simulink model "HexrotorDynamicModel_matlab2010"  (Simulink 7.6)
settings: Solver=ode3  SolverMode=SingleTasking  StartTime=0.0  StopTime=20  FixedStep=0.0005  RelTol=1e-3
values from neighbouring files (symbols this model uses):
  alpha = pi/180 * 13.6    (= 0.237364778271)    [IdealParameter.m]    (also in ParLuk11.m = deg2rad(13.6); Parameter.m = [-alpha_i;alpha_i;-alpha_i;alpha_i;-alpha_i;alpha_i]; ParameterIdeal.m = [-alpha_i;alpha_i;-alpha_i;alpha_i;-alpha_i;alpha_i]; ParameterVIVE.m = [alpha_i;-alpha_i;alpha_i;-alpha_i;alpha_i;-alpha_i])
  alpha_0 = alpha    (= 0.237364778271)    [IdealParameter.m]    (also in Parameter.m = alpha; ParameterIdeal.m = alpha*1.01; ParameterVIVE.m = alpha*1.01; ParameterVO.m = alpha*1.01)
  angular_noise = 0    [IdealParameter.m]    (also in Parameter.m = 0.5; ParameterIdeal.m; ParameterVIVE.m; ParameterVO.m)
  b = 1.1e-06    [IdealParameter.m]    (also in ParLuk11.m = 1.14e-07; Parameter.m = 8.944e-07; ParameterIdeal.m; ParameterVIVE.m)
  b_0 = b*1.15    (= 1.265e-06)    [IdealParameter.m]    (also in Parameter.m = 8.944e-07; ParameterIdeal.m; ParameterVIVE.m; ParameterVO.m)
  beta = 0    [IdealParameter.m]    (also in ParLuk11.m; Parameter.m = [beta_i; beta_i; beta_i; beta_i; beta_i; beta_i]; ParameterIdeal.m = [beta_i; beta_i; beta_i; beta_i; beta_i; beta_i]; ParameterVIVE.m = [beta_i; beta_i; beta_i; beta_i; beta_i; beta_i])
  beta_0 = beta    (= 0)    [IdealParameter.m]    (also in Parameter.m = beta; ParameterIdeal.m = beta*0.99; ParameterVIVE.m = beta*0.99; ParameterVO.m = beta*0.99)
  eta = 1    [Controllability.m]    (also in IdealParameter.m = 75; Parameter.m = 2; ParameterIdeal.m = 40; ParameterVIVE.m = 10)
  eta_rot = 50    [IdealParameter.m]    (also in Parameter.m = 2; ParameterIdeal.m = 20; ParameterVIVE.m = 5; ParameterVO.m = 2)
  g = 9.81    [IdealParameter.m]    (also in ParLuk11.m; Parameter.m; ParameterIdeal.m; ParameterVIVE.m)
  g_0 = g*0.99    (= 9.7119)    [IdealParameter.m]    (also in Parameter.m = 9.81; ParameterIdeal.m = 9.81; ParameterVIVE.m = 9.81; ParameterVO.m = 9.81)
  IB = [Ixx 0 0; 0 Iyy 0; 0 0 Izz]    [IdealParameter.m]    (also in ParLuk11.m; Parameter.m; ParameterIdeal.m; ParameterVIVE.m)
  IB_0 = IB*1.07    [IdealParameter.m]    (also in Parameter.m = IB; ParameterIdeal.m; ParameterVIVE.m; ParameterVO.m)
  k = 5.6e-05    [IdealParameter.m]    (also in ParLuk11.m = 2.98e-06; Parameter.m = 4.472e-05; ParameterIdeal.m; ParameterVIVE.m = 5.13e-05)
  K_0 = Ts/(T_rotor_0+Ts)    (= 0.0384615384615)    [IdealParameter.m]    (also in Parameter.m = 0.230769230769; ParameterIdeal.m; ParameterVIVE.m = 0.0350877192982; ParameterVO.m = 0.214285714286)
  k_0 = k*1.16    (= 6.496e-05)    [IdealParameter.m]    (also in Parameter.m = 4.472e-05; ParameterIdeal.m; ParameterVIVE.m = 5.9508e-05; ParameterVO.m)
  K_d = diag([5,5,5,2,2,2])    [ParLuk11.m]
  K_p1 = 10*eye(3)    [ParLuk11.m]
  k_p2 = 3    [ParLuk11.m]
  K_P_1 = 15*eye(3)    [IdealParameter.m]    (also in Parameter.m = 2*eye(3); ParameterIdeal.m; ParameterVIVE.m = 10*eye(3); ParameterVO.m = 2*eye(3))
  K_P_2 = 50*eye(3)    [IdealParameter.m]    (also in Parameter.m = 4*eye(3); ParameterIdeal.m; ParameterVIVE.m = 10*eye(3); ParameterVO.m = 4*eye(3))
  K_P_3 = 60*eye(3)    [IdealParameter.m]    (also in Parameter.m = 6*eye(3); ParameterIdeal.m; ParameterVIVE.m = 10*eye(3); ParameterVO.m = 6*eye(3))
  K_P_D = 30*eye(3)    [IdealParameter.m]    (also in ParLuk11.m = 10*eye(3); Parameter.m = 5*eye(3); ParameterIdeal.m; ParameterVIVE.m = 15*eye(3))
  K_P_I = 100*eye(3)    [IdealParameter.m]    (also in ParLuk11.m = 10*eye(3); Parameter.m = 10*eye(3); ParameterIdeal.m = 80*eye(3); ParameterVIVE.m)
  K_P_P = 100*eye(3)    [IdealParameter.m]    (also in ParLuk11.m = 20*eye(3); Parameter.m = 10*eye(3); ParameterIdeal.m = 130*eye(3); ParameterVIVE.m)
  K_R_1 = 40*eye(3)    [IdealParameter.m]    (also in Parameter.m = 2*eye(3); ParameterIdeal.m; ParameterVIVE.m = 10*eye(3); ParameterVO.m = 2*eye(3))
  K_R_2 = 100*eye(3)    [IdealParameter.m]    (also in Parameter.m = 4*eye(3); ParameterIdeal.m; ParameterVIVE.m = 10*eye(3); ParameterVO.m = 4*eye(3))
  K_R_3 = 50*eye(4)    [IdealParameter.m]    (also in Parameter.m = 6*eye(4); ParameterIdeal.m; ParameterVIVE.m = 10*eye(4); ParameterVO.m = 6*eye(4))
  K_R_D = 30*eye(3)    [IdealParameter.m]    (also in ParLuk11.m = 10*eye(3); Parameter.m = 5*eye(3); ParameterIdeal.m; ParameterVIVE.m = 15*eye(3))
  K_R_I = 100*eye(3)    [IdealParameter.m]    (also in ParLuk11.m = 10*eye(3); Parameter.m = 10*eye(3); ParameterIdeal.m = 80*eye(3); ParameterVIVE.m)
  K_R_P = 100*eye(3)    [IdealParameter.m]    (also in ParLuk11.m = 20*eye(3); Parameter.m = 10*eye(3); ParameterIdeal.m = 130*eye(3); ParameterVIVE.m)
  L = 0.4    [IdealParameter.m]    (also in ParLuk11.m = 1; Parameter.m; ParameterIdeal.m; ParameterVIVE.m = 0.6)
  L_0 = L*1.02    (= 0.408)    [IdealParameter.m]    (also in Parameter.m = 0.4; ParameterIdeal.m; ParameterVIVE.m = 0.612; ParameterVO.m)
  lambda = 10    [IdealParameter.m]    (also in Parameter.m = 3; ParameterIdeal.m = 5; ParameterVIVE.m = 5; ParameterVO.m = 3)
  lambda_rot = 10    [IdealParameter.m]    (also in Parameter.m = 3; ParameterIdeal.m; ParameterVIVE.m = 5; ParameterVO.m = 3)
  m = 1    [Controllability.m]    (also in IdealParameter.m = 2.5; ParLuk11.m = 0.6; Parameter.m = 4.85; ParameterIdeal.m = 4.85)
  M = 50    [IdealParameter.m]    (also in Parameter.m = 6; ParameterIdeal.m = 100; ParameterVIVE.m = 5; ParameterVO.m = 6)
  m_0 = m*1.03    (= 2.575)    [IdealParameter.m]    (also in Parameter.m = 4.85; ParameterIdeal.m = 4.9955; ParameterVIVE.m = 4.52994; ParameterVO.m = 4.9955)
  M_rot = 50    [IdealParameter.m]    (also in Parameter.m = 6; ParameterIdeal.m = 15; ParameterVIVE.m = 1; ParameterVO.m = 6)
  omega_noise = 0    [IdealParameter.m]    (also in Parameter.m = sqrt(2)*angular_noise/Ts * pi/180; ParameterIdeal.m; ParameterVIVE.m; ParameterVO.m)
  p_noise = 0    [IdealParameter.m]    (also in Parameter.m = 0.001; ParameterIdeal.m; ParameterVIVE.m; ParameterVO.m)
  T_delay = 0    [IdealParameter.m]    (also in Parameter.m = 0.1; ParameterIdeal.m; ParameterVIVE.m = 0.04; ParameterVO.m = 0.1)
  T_rotor = 0.1    [IdealParameter.m]    (also in Parameter.m; ParameterIdeal.m; ParameterVIVE.m; ParameterVO.m)
  Ts = 1/250    (= 0.004)    [IdealParameter.m]    (also in Parameter.m = 0.03; ParameterIdeal.m; ParameterVIVE.m; ParameterVO.m = 0.03)
  v_noise = 0    [IdealParameter.m]    (also in Parameter.m = sqrt(2)*p_noise/Ts; ParameterIdeal.m; ParameterVIVE.m; ParameterVO.m)
  z_p_0 = T_rotor_0/(T_rotor_0+Ts)    (= 0.961538461538)    [IdealParameter.m]    (also in Parameter.m = 0.769230769231; ParameterIdeal.m; ParameterVIVE.m = 0.964912280702; ParameterVO.m = 0.785714285714)
undefined symbols (not defined in the file or in its folder): DiscIntNeverNeededParam, k_ad, k_ap, k_pd, k_pp, k_z
libraries: vrlib x8, simulink x7, dspmtrx3 x3
(part 1 of 3)
settings Model: Creator=jan  LastModifiedBy=Jan  CovMetricSettings=dwe  CovHtmlReporting=off  covSaveCumulativeToWorkspaceVar=off  CovSaveSingleToWorkspaceVar=off  CovExternalEMLEnable=on
settings DataIOCC: LimitDataPoints=off  SaveFormat=StructureWithTime
settings OptimizationCC: ExpressionDepthLimit=128
settings DebuggingCC: UnderspecifiedInitializationDetection=Simplified  MergeDetectMultiDrivingBlocksExec=error  SolverPrmCheckMsg=none  FcnCallInpInsideContextMsg=Enable All  StateNameClashWarn=none  SFUnexpectedBacktrackingDiag=error  SFNoUnconditionalDefaultTransitionDiag=error
settings HardwareCC: ProdBitPerPointer=64  ProdLargestAtomicFloat=Float  ProdIntDivRoundTo=Zero  ProdEndianess=LittleEndian  ProdHWDeviceType=Specified
settings CodeAppCC: CustomSymbolStrType=$N$R$M_T
settings GRTTargetCC: TargetFunctionLibrary=C99 (ISO)  GeneratePreprocessorConditionals=Use local settings

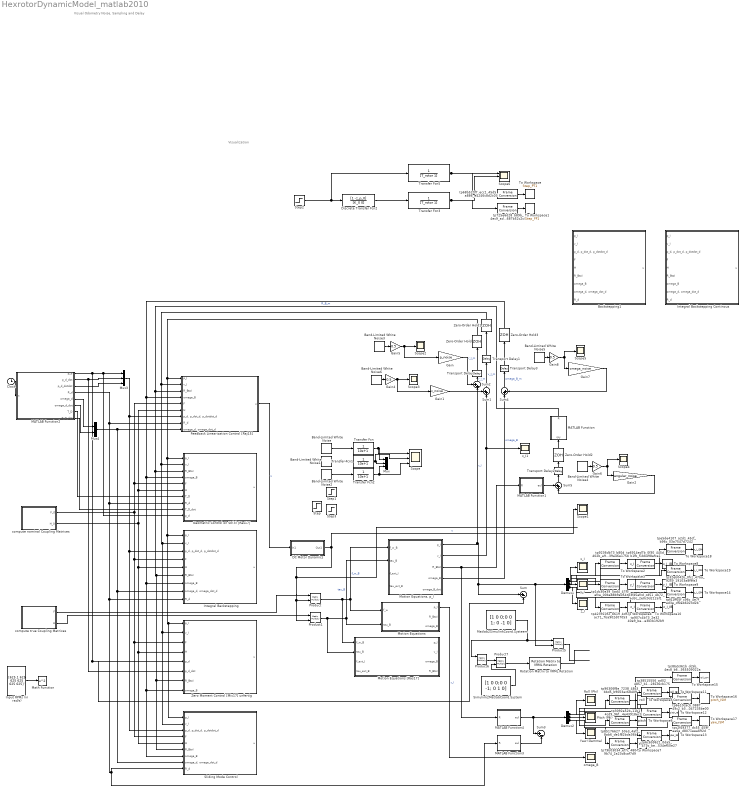
== system HexrotorDynamicModel_matlab2010 ==
  note: Visual Odometry Noise, Sampling and Delay
  note: Visualization
  Backstepping1 : Subsystem
  Band-Limited White Noise : simulink/Sources/Band-Limited White Noise  Cov=10  Ts=0.1  seed=[28341]  VectorParams1D=off
  Band-Limited White Noise1 : simulink/Sources/Band-Limited White Noise  Cov=10  Ts=0.1  seed=[23342]  VectorParams1D=off
  Band-Limited White Noise2 : simulink/Sources/Band-Limited White Noise  Cov=10  Ts=0.1  seed=[23441]  VectorParams1D=off
  Band-Limited White Noise3 : simulink/Sources/Band-Limited White Noise  Cov=[0.01; 0.01; 0.01]  Ts=Ts  seed=[22352; 29655; 12541]  VectorParams1D=off
  Band-Limited White Noise4 : simulink/Sources/Band-Limited White Noise  Cov=[0.01; 0.01; 0.01]  Ts=Ts  seed=[11351; 22653; 52546]  VectorParams1D=off
  Band-Limited White Noise5 : simulink/Sources/Band-Limited White Noise  Cov=[0.01; 0.01; 0.01]  Ts=Ts  seed=[12451; 82653; 82546]  VectorParams1D=off
  Band-Limited White Noise6 : simulink/Sources/Band-Limited White Noise  Cov=[0.01; 0.01; 0.01]  Ts=Ts  seed=[22351; 29653; 12546]  VectorParams1D=off
  Clock : Clock
  "DC Motor Dynamics " : Subsystem  TreatAsAtomicUnit=on
  Demux1 : Demux  Outputs=3
  Demux2 : Demux  Outputs=3
  Discrete Transfer Fcn2 : DiscreteTransferFcn  Numerator=[1 -z_p_0]  Denominator=[K_0 0]  InitialStates=550  SampleTime=Ts
  Feedback Linearization Control [Raj15] : Subsystem
  Gain : Gain  Gain=p_noise
  Gain1 : Gain  Gain=v_noise
  Gain2 : Gain  Gain=angular_noise
  Gain{4..6,8} (4 alike) : Gain  Gain=0.5
  Gain7 : Gain  Gain=omega_noise
  Geometric Control on SE(3) [Ras17] : Subsystem
  Input RPMs (in rad/s) : Constant  Value=[625.1 625 625 625 625 625]'  VectorParams1D=off
  Integral Backstepping : Subsystem
  "Integral Backstepping Continous " : Subsystem
  MATLAB Function : Stateflow chart  TreatAsAtomicUnit=on
      settings: PermitHierarchicalResolution=ParametersOnly
  MATLAB Function1 : Stateflow chart  TreatAsAtomicUnit=on
      settings: PermitHierarchicalResolution=ParametersOnly
  MATLAB Function2 : Stateflow chart  TreatAsAtomicUnit=on
      settings: PermitHierarchicalResolution=ParametersOnly
  MATLAB Function3 : Stateflow chart  TreatAsAtomicUnit=on
      settings: PermitHierarchicalResolution=ParametersOnly
  MATLAB Function4 : Stateflow chart  TreatAsAtomicUnit=on
      settings: PermitHierarchicalResolution=ParametersOnly
  Math Function : Math  Operator=square  SaturateOnIntegerOverflow=on
  "Matlab2SimulinkCoord.Systeem " : Constant  Value=[1 0 0;0 0 1; 0 -1 0]  VectorParams1D=off
  Motion Equations : Subsystem
  Motion Equations [Ras17] : Subsystem
  "Motion Equations, p_I" : Subsystem
  Mux : Mux  Inputs=3
  Mux3 : Mux  Inputs=3
  Mux4 : Mux  Inputs=2
  Pitch (Psi) : Scope
      settings: TimeRange=auto  MaxDataPoints=5000  SaveToWorkspace=off  YMin=-3.22277  YMax=12.55112  SampleTime=-1
  Product{,1,5..7} (5 alike) : Product  Multiplication=Matrix(*)
  Roll (Phi) : Scope
      settings: TimeRange=auto  MaxDataPoints=5000  SaveToWorkspace=off  SaveName=ScopeData2  YMin=-4.01127  YMax=16.26235  SampleTime=-1
  Rotation Matrix to VRML Rotation : vrlib/Utilities/Rotation Matrix to VRML Rotation  maxzero=1e-12
  Scope : Scope  NumInputPorts=3
      settings: TimeRange=auto  MaxDataPoints=5000  SaveToWorkspace=off  YMin=-1.78932~-5~-5  YMax=1.08657~5~5  SampleTime=-1
  Scope{1..5} (5 alike) : Scope
      Scope1 settings: TimeRange=auto  MaxDataPoints=5000  SaveToWorkspace=off  YMin=-244096.59135  YMax=3111530.80524  SampleTime=-1
      Scope2 settings: TimeRange=auto  MaxDataPoints=5000  SaveToWorkspace=off  YMin=-1.60588  YMax=1.50821  SampleTime=-1
      Scope3 settings: TimeRange=auto  MaxDataPoints=5000  SaveToWorkspace=off  SaveName=ScopeData2  YMin=-1.55633  YMax=1.34059  SampleTime=-1
      Scope4 settings: TimeRange=auto  MaxDataPoints=5000  SaveToWorkspace=off  SaveName=ScopeData2  YMin=-1.57808  YMax=1.44255  SampleTime=-1
      Scope5 settings: TimeRange=auto  MaxDataPoints=5000  SaveToWorkspace=off  SaveName=ScopeData3  YMin=-3.75052  YMax=3.91407  SampleTime=-1
  Scope6 : Scope  NumInputPorts=3
      settings: TimeRange=auto  MaxDataPoints=5000  SaveToWorkspace=off  YMin=-0.61685~-5~-5  YMax=2.28631~5~5  SampleTime=-1
  "Simulink2MatlabCoord.System " : Constant  Value=[1 0 0;0 0 -1; 0 1 0]  VectorParams1D=off
  Sliding Mode Control : Subsystem
  Step : Step  Time=0.1  Before=[6,0,6]'  After=[0,0,0]'  SampleTime=0  VectorParams1D=off
  Step1 : Step  Before=[0;0;0]  After=[10;1;1]  SampleTime=0  VectorParams1D=off
  Step2 : Step  SampleTime=0
  Step3 : Step  Before=[0;0;0]  After=[5;1;1]  SampleTime=0  VectorParams1D=off
  Sum : Sum  Inputs=|+-
  Sum1 : Sum  Inputs=++|
  Sum2 : Sum  Inputs=++|
  Sum3 : Sum  Inputs=|+-
  Sum4 : Sum  Inputs=|++
  Sum5 : Sum  Inputs=++|
  To Workspace : ToWorkspace  VariableName=Step_PT1  SampleTime=Ts
  To Workspace1 : ToWorkspace  VariableName=Step_FF1  SampleTime=Ts
  To Workspace10 : ToWorkspace  VariableName=z_I_IB  SampleTime=Ts
  To Workspace11 : ToWorkspace  VariableName=roll_IB  SampleTime=Ts
  To Workspace12 : ToWorkspace  VariableName=pitch_IB  SampleTime=Ts
  To Workspace13 : ToWorkspace  VariableName=yaw_IB  SampleTime=Ts
  To Workspace14 : ToWorkspace  VariableName=z_I_ISM  SampleTime=Ts
  To Workspace15 : ToWorkspace  VariableName=roll_ISM  SampleTime=Ts
  To Workspace16 : ToWorkspace  VariableName=pitch_ISM  SampleTime=Ts
  To Workspace17 : ToWorkspace  VariableName=yaw_ISM  SampleTime=Ts
  To Workspace18 : ToWorkspace  VariableName=x_I_ISM  SampleTime=Ts
  To Workspace19 : ToWorkspace  VariableName=y_I_ISM  SampleTime=Ts
  To Workspace2 : ToWorkspace  VariableName=x_I  SampleTime=Ts
  To Workspace3 : ToWorkspace  VariableName=y_I  SampleTime=Ts
  To Workspace4 : ToWorkspace  VariableName=z_I  SampleTime=Ts
  To Workspace5 : ToWorkspace  VariableName=roll  SampleTime=Ts
  To Workspace6 : ToWorkspace  VariableName=pitch  SampleTime=Ts
  To Workspace7 : ToWorkspace  VariableName=yaw  SampleTime=Ts
  To Workspace8 : ToWorkspace  VariableName=x_I_IB  SampleTime=Ts
  To Workspace9 : ToWorkspace  VariableName=y_I_IB  SampleTime=Ts
  Transfer Fcn : TransferFcn  Denominator=[10 1]
  Transfer Fcn1 : TransferFcn  Denominator=[10 1]
  Transfer Fcn2 : TransferFcn  Denominator=[10 1]
  Transfer Fcn3 : TransferFcn  Denominator=[T_rotor 1]
  Transfer Fcn5 : TransferFcn  Denominator=[T_rotor 1]
  Transport Delay{,1..3} (4 alike) : TransportDelay  DelayTime=T_delay  InitialOutput=[0;0;0]
  Yaw (Gamma) : Scope
      settings: TimeRange=auto  MaxDataPoints=5000  SaveToWorkspace=off  SaveName=ScopeData3  YMin=-2.81636  YMax=2.98602  SampleTime=-1
  Zero Moment Control [Mic17] unfertig : Subsystem
  Zero-Order Hold : ZeroOrderHold  SampleTime=0.02
  Zero-Order Hold1 : ZeroOrderHold  SampleTime=0.01
  Zero-Order Hold2 : ZeroOrderHold  SampleTime=Ts
  Zero-Order Hold3 : ZeroOrderHold  SampleTime=0.01
  compute nominal Coupling Matrices : Subsystem
  compute true Coupling Matrices : Subsystem
  omega_B : Scope
      settings: TimeRange=auto  LimitDataPoints=on  MaxDataPoints=5000  SaveToWorkspace=off  SaveName=ScopeData4  YMin=-0.00000000000000000  YMax=0.00000000000000017  SampleTime=-1  DataFormat=Array
  tp1dc30e39_5ad4_47f3_afca_00ba88b9e054 : FrameConversion  InheritSamplingMode=off  OutFrame=Sample-based
  tp3092a52b_11b1_4cd9_96f5_a04e43918ec3 : FrameConversion  InheritSamplingMode=off  OutFrame=Sample-based
  tp32eb042b_0fcc_47ba_92c9_19103a8f9fa3 : FrameConversion  InheritSamplingMode=off  OutFrame=Sample-based
  tp38515556_ad02_4857_b18b_e4281c6cb175 : FrameConversion  InheritSamplingMode=off  OutFrame=Sample-based
  tp38a5361b_dc5b_4ec8_b600_69955509022a : FrameConversion  InheritSamplingMode=off  OutFrame=Sample-based
  tp3f45afcd_cd51_4b72_ad3c_2e0c0d212af1 : FrameConversion  InheritSamplingMode=off  OutFrame=Sample-based
  tp4239105c_b619_4df0_ac71_7ba902d07053 : FrameConversion  InheritSamplingMode=off  OutFrame=Sample-based
  tp68b520f7_ecc1_45d5_a886_e4246c8d2c03 : FrameConversion  InheritSamplingMode=off  OutFrame=Sample-based
  tp6914ed7b_0f30_445d_b1fb_f1bb498efca1 : FrameConversion  InheritSamplingMode=off  OutFrame=Sample-based
  tp6c6b9621_0da5_473c_be95_13534ef50e27 : FrameConversion  InheritSamplingMode=off  OutFrame=Sample-based
  tp6e10cacb_0887_49c2_b351_a1047235be00 : FrameConversion  InheritSamplingMode=off  OutFrame=Sample-based
  tp725e6d28_b89b_4ec9_adef_fa687b52c2c8 : FrameConversion  InheritSamplingMode=off  OutFrame=Sample-based
  tp79b03034_ef7c_4804_9b74_2a23c8caf7d9 : FrameConversion  InheritSamplingMode=off  OutFrame=Sample-based
  tp85176627_50a3_4af2_8ab6_de1f82bda36b : FrameConversion  InheritSamplingMode=off  OutFrame=Sample-based
  tp907c4b73_2e32_40e9_be19_e2e3bcb192b9 : FrameConversion  InheritSamplingMode=off  OutFrame=Sample-based
  tp9236db73_b80d_402b_a970_1639a46e175b : FrameConversion  InheritSamplingMode=off  OutFrame=Sample-based
  tp96306f8e_7238_48c3_bbd5_b9003ac68409 : FrameConversion  InheritSamplingMode=off  OutFrame=Sample-based
  tpc2f49377_dc55_459f_aa6e_d8071eeab92d : FrameConversion  InheritSamplingMode=off  OutFrame=Sample-based
  tpe5de4107_a2d1_45cf_b96c_03a7547d7242 : FrameConversion  InheritSamplingMode=off  OutFrame=Sample-based
  tpf41ff05f_c96c_4e7f_ad3e_df0ab6023d2b : FrameConversion  InheritSamplingMode=off  OutFrame=Sample-based
  x_I : Scope
      settings: TimeRange=auto  MaxDataPoints=5000  SaveToWorkspace=off  SaveName=ScopeData6  YMin=-0.2003  YMax=1.67814  SampleTime=-1
  x_I1 : Scope
      settings: TimeRange=auto  MaxDataPoints=5000  SaveToWorkspace=off  YMin=-0.67724  YMax=1.12529  SampleTime=-1
  y_I : Scope
      settings: TimeRange=auto  MaxDataPoints=5000  SaveToWorkspace=off  SaveName=ScopeData7  YMin=-0.14547  YMax=1.20694  SampleTime=-1
  z_I : Scope
      settings: TimeRange=auto  MaxDataPoints=5000  SaveToWorkspace=off  SaveName=ScopeData  YMin=-0.17063  YMax=0.10776  SampleTime=-1
  wires:
  Product6/1 -> Product7/1
  Product5/1 -> ?
  Demux2/2 -> tp3092a52b_11b1_4cd9_96f5_a04e43918ec3/1, tp6e10cacb_0887_49c2_b351_a1047235be00/1, Pitch (Psi)/1, tp85176627_50a3_4af2_8ab6_de1f82bda36b/1
  Input RPMs (in rad/s)/1 -> Math Function/1
  Transport Delay/1 -> Zero-Order Hold/1  "r_I_m"
  Demux1/3 -> tp907c4b73_2e32_40e9_be19_e2e3bcb192b9/1, tpf41ff05f_c96c_4e7f_ad3e_df0ab6023d2b/1, z_I/1, tp4239105c_b619_4df0_ac71_7ba902d07053/1
  Demux1/1 -> tpe5de4107_a2d1_45cf_b96c_03a7547d7242/1, tp9236db73_b80d_402b_a970_1639a46e175b/1, x_I/1, tp6914ed7b_0f30_445d_b1fb_f1bb498efca1/1
  "DC Motor Dynamics "/1(Out1) -> Product1/2, Product/2, Scope1/1  "u"
  Demux1/2 -> tp32eb042b_0fcc_47ba_92c9_19103a8f9fa3/1, tp1dc30e39_5ad4_47f3_afca_00ba88b9e054/1, y_I/1, tp3f45afcd_cd51_4b72_ad3c_2e0c0d212af1/1
  Rotation Matrix to VRML Rotation/1 -> ?
  Demux2/1 -> tp38515556_ad02_4857_b18b_e4281c6cb175/1, tp38a5361b_dc5b_4ec8_b600_69955509022a/1, Roll (Phi)/1, tp96306f8e_7238_48c3_bbd5_b9003ac68409/1
  "Matlab2SimulinkCoord.Systeem "/1 -> Product6/1, Product5/1
  Product7/1 -> Rotation Matrix to VRML Rotation/1
  "Simulink2MatlabCoord.System "/1 -> Product7/2
  MATLAB Function/1(R) -> Geometric Control on SE(3) [Ras17]/3("R_BtoI "), Sliding Mode Control/6(R_BtoI), Zero Moment Control [Mic17] unfertig/7(R_BtoI), Integral Backstepping/6(R_BtoI), Feedback Linearization Control [Raj15]/3("R_BtoI ")  "R_B_m"
  Sum4/1 -> Transport Delay3/1  "omega_B_m"
  Motion Equations/1(p_I) -> omega_B/1  "r_I"
  compute nominal Coupling Matrices/1(F_0) -> Sliding Mode Control/4(F), Zero Moment Control [Mic17] unfertig/3(F), Integral Backstepping/4(F), Geometric Control on SE(3) [Ras17]/5(F), Feedback Linearization Control [Raj15]/5(F)
  Product/1 -> Motion Equations [Ras17]/1("f_w_B "), Motion Equations/1("f_w "), "Motion Equations, p_I"/1("f_w_B ")  "f_w_B"
  compute nominal Coupling Matrices/2("H_0 ") -> Zero Moment Control [Mic17] unfertig/4(H), Sliding Mode Control/5(H), Integral Backstepping/5(H), Geometric Control on SE(3) [Ras17]/6(H), Feedback Linearization Control [Raj15]/6(H)
  Product1/1 -> Motion Equations [Ras17]/2(tau_B), "Motion Equations, p_I"/2(tau_B), Motion Equations/2(tau_B)  "tau_B"
  Clock/1 -> MATLAB Function2/1(t)
  MATLAB Function2/3(p_d_dotdot) -> Mux3/3
  MATLAB Function2/2(p_d_dot) -> Zero Moment Control [Mic17] unfertig/6(p_d_dot), Mux3/2
  MATLAB Function2/1(p_d) -> Sum/2, Zero Moment Control [Mic17] unfertig/5(p_d), Geometric Control on SE(3) [Ras17]/10(p_d), Mux3/1
  MATLAB Function2/6(omega_d_dot) -> Mux4/2
  Band-Limited White Noise/1 -> Transfer Fcn/1
  Transfer Fcn/1 -> Scope/1, Mux/1
  Transfer Fcn2/1 -> Scope/3, Mux/3
  Band-Limited White Noise1/1 -> Transfer Fcn1/1
  Band-Limited White Noise2/1 -> Transfer Fcn2/1
  Transfer Fcn1/1 -> Scope/2, Mux/2
  Mux3/1 -> Sliding Mode Control/3("p_d, p_dot_d, p_dotdot_d"), Integral Backstepping/3("p_d, p_dot_d, p_dotdot_d"), Feedback Linearization Control [Raj15]/7("p_d, p_dot_d, p_dotdot_d")
  MATLAB Function2/4(R_d) -> MATLAB Function3/1(R), Sliding Mode Control/9(R_d), Integral Backstepping/9(R_d), Geometric Control on SE(3) [Ras17]/8(R_d), Feedback Linearization Control [Raj15]/8(R_d)
  MATLAB Function2/5(omega_d) -> Mux4/1
  Mux4/1 -> Sliding Mode Control/8("omega_d, omega_dot_d"), Integral Backstepping/8("omega_d, omega_dot_d"), Feedback Linearization Control [Raj15]/9("omega_d, omega_dot_d")
  MATLAB Function2/7(T_D) -> Geometric Control on SE(3) [Ras17]/7(T_D)
  MATLAB Function2/8(T_D_dot) -> Geometric Control on SE(3) [Ras17]/9(T_D_dot)
  compute true Coupling Matrices/1(F) -> Product/1
  compute true Coupling Matrices/2(H) -> Product1/1
  "Motion Equations, p_I"/1(p_I) -> Sum/1, Demux1/1, Product5/2, Sum2/2  "r_I"
  "Motion Equations, p_I"/2(v_I) -> x_I1/1, Sum1/2
  "Motion Equations, p_I"/3(R_BtoI) -> MATLAB Function4/1(R), MATLAB Function1/1(R)
  "Motion Equations, p_I"/4(omega_B) -> Sum4/1  "omega_B"
  Gain/1 -> Sum2/1
  Band-Limited White Noise3/1 -> Gain5/1
  Gain4/1 -> Gain1/1, Scope3/1
  Gain1/1 -> Sum1/1
  Sum2/1 -> Transport Delay/1  "r_I_m"
  Transport Delay1/1 -> Zero-Order Hold1/1
  Sum1/1 -> Transport Delay1/1  "v_I_m"
  Zero-Order Hold/1 -> Geometric Control on SE(3) [Ras17]/1("p_I "), Sliding Mode Control/1(p_I), Zero Moment Control [Mic17] unfertig/1(p_I), Integral Backstepping/1(p_I), Feedback Linearization Control [Raj15]/1("p_I ")
  Zero-Order Hold1/1 -> Sliding Mode Control/2(v_I), Zero Moment Control [Mic17] unfertig/2(v_I), Integral Backstepping/2(v_I), Geometric Control on SE(3) [Ras17]/2(v_I), Feedback Linearization Control [Raj15]/2(v_I)
  MATLAB Function1/1(eul) -> Sum5/1
  Gain6/1 -> Scope4/1, Gain2/1
  Sum5/1 -> Transport Delay2/1
  Gain2/1 -> Sum5/2
  Zero-Order Hold2/1 -> MATLAB Function/1(rpy)
  Transport Delay2/1 -> Zero-Order Hold2/1
  Transport Delay3/1 -> Zero-Order Hold3/1
  Zero-Order Hold3/1 -> Sliding Mode Control/7(omega_B), Zero Moment Control [Mic17] unfertig/8(omega_B), Integral Backstepping/7(omega_B), Geometric Control on SE(3) [Ras17]/4(omega_B), Feedback Linearization Control [Raj15]/4(omega_B)
  Feedback Linearization Control [Raj15]/1(u) -> "DC Motor Dynamics "/1(In1)  "u"
  Band-Limited White Noise6/1 -> Gain4/1
  Gain5/1 -> Gain/1, Scope2/1
  Band-Limited White Noise4/1 -> Gain6/1
  Gain8/1 -> Scope5/1, Gain7/1
  Band-Limited White Noise5/1 -> Gain8/1
  Gain7/1 -> Sum4/2
  Transfer Fcn3/1 -> Scope6/2, tp725e6d28_b89b_4ec9_adef_fa687b52c2c8/1
  Step2/1 -> Transfer Fcn5/1, Discrete Transfer Fcn2/1
  Discrete Transfer Fcn2/1 -> Transfer Fcn3/1
  Transfer Fcn5/1 -> Scope6/1, tp68b520f7_ecc1_45d5_a886_e4246c8d2c03/1
  Demux2/3 -> tp6c6b9621_0da5_473c_be95_13534ef50e27/1, tpc2f49377_dc55_459f_aa6e_d8071eeab92d/1, Yaw (Gamma)/1, tp79b03034_ef7c_4804_9b74_2a23c8caf7d9/1
  MATLAB Function3/1(eul) -> Sum3/2
  MATLAB Function4/1(eul) -> Demux2/1, Sum3/1
  tp68b520f7_ecc1_45d5_a886_e4246c8d2c03/1 -> To Workspace/1
  tp725e6d28_b89b_4ec9_adef_fa687b52c2c8/1 -> To Workspace1/1
  tp907c4b73_2e32_40e9_be19_e2e3bcb192b9/1 -> To Workspace10/1
  tp38515556_ad02_4857_b18b_e4281c6cb175/1 -> To Workspace11/1
  tp3092a52b_11b1_4cd9_96f5_a04e43918ec3/1 -> To Workspace12/1
  tp6c6b9621_0da5_473c_be95_13534ef50e27/1 -> To Workspace13/1
  tpf41ff05f_c96c_4e7f_ad3e_df0ab6023d2b/1 -> To Workspace14/1
  tp38a5361b_dc5b_4ec8_b600_69955509022a/1 -> To Workspace15/1
  tp6e10cacb_0887_49c2_b351_a1047235be00/1 -> To Workspace16/1
  tpc2f49377_dc55_459f_aa6e_d8071eeab92d/1 -> To Workspace17/1
  tpe5de4107_a2d1_45cf_b96c_03a7547d7242/1 -> To Workspace18/1
  tp32eb042b_0fcc_47ba_92c9_19103a8f9fa3/1 -> To Workspace19/1
  tp9236db73_b80d_402b_a970_1639a46e175b/1 -> To Workspace2/1
  tp1dc30e39_5ad4_47f3_afca_00ba88b9e054/1 -> To Workspace3/1
  tp4239105c_b619_4df0_ac71_7ba902d07053/1 -> To Workspace4/1
  tp96306f8e_7238_48c3_bbd5_b9003ac68409/1 -> To Workspace5/1
  tp85176627_50a3_4af2_8ab6_de1f82bda36b/1 -> To Workspace6/1
  tp79b03034_ef7c_4804_9b74_2a23c8caf7d9/1 -> To Workspace7/1
  tp6914ed7b_0f30_445d_b1fb_f1bb498efca1/1 -> To Workspace8/1
  tp3f45afcd_cd51_4b72_ad3c_2e0c0d212af1/1 -> To Workspace9/1

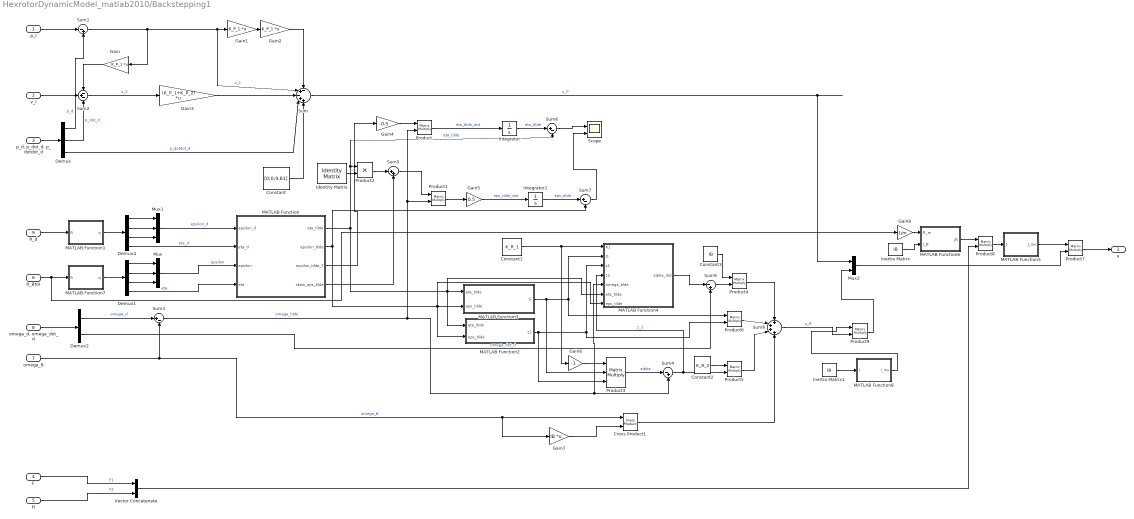
== system HexrotorDynamicModel_matlab2010/Backstepping1 ==
  p_I : Inport
  v_I : Inport  Port=2
  "p_d, p_dot_d, p_dotdot_d" : Inport  Port=3
  F : Inport  Port=4
  H : Inport  Port=5
  R_BtoI : Inport  Port=6
  omega_B : Inport  Port=7
  "omega_d, omega_dot_d" : Inport  Port=8
  R_d : Inport  Port=9
  Constant : Constant  Value=[0;0;9.81]  VectorParams1D=off
  Constant1 : Constant  Value=K_R_1  VectorParams1D=off
  Constant2 : Constant  Value=K_R_2  VectorParams1D=off
  Constant3 : Constant  Value=IB  VectorParams1D=off
  Cross Product1 : vrlib/Utilities/Cross Product
  Demux : Demux  Outputs=3
  Demux1 : Demux
  Demux2 : Demux  Outputs=2
  Demux4 : Demux
  Gain : Gain  Gain=K_P_1  Multiplication=Matrix(K*u)
  Gain1 : Gain  Gain=K_P_1  Multiplication=Matrix(K*u)
  Gain2 : Gain  Gain=K_P_1  Multiplication=Matrix(K*u)
  Gain3 : Gain  Gain=(K_P_1+K_P_2)  Multiplication=Matrix(K*u)
  Gain4 : Gain  Gain=-0.5
  Gain5 : Gain  Gain=0.5
  Gain6 : Gain  Gain=-1
  Gain7 : Gain  Gain=IB  Multiplication=Matrix(K*u)
  Gain8 : Gain  Gain=1/m
  Identity Matrix : dspmtrx3/Identity Matrix  Inherit=off  N=3  Ts=inf  dataType=double  isSigned=on  wordLen=16  udDataType=sfix(16)  fracBitsMode=Best precision  numFracBits=15  OutDataTypeStr=double  LastOutDataTypeStr=double
  Inertia Matrix : Constant  Value=IB  VectorParams1D=off
  Inertia Matrix1 : Constant  Value=IB  VectorParams1D=off
  Integrator : Integrator  InitialCondition=1
  Integrator1 : Integrator  InitialCondition=[0;0;0]
  MATLAB Function : Stateflow chart  TreatAsAtomicUnit=on
      settings: PermitHierarchicalResolution=ParametersOnly
  MATLAB Function1 : Stateflow chart  TreatAsAtomicUnit=on
      settings: PermitHierarchicalResolution=ParametersOnly
  MATLAB Function2 : Stateflow chart  TreatAsAtomicUnit=on
      settings: PermitHierarchicalResolution=ParametersOnly
  MATLAB Function3 : Stateflow chart  TreatAsAtomicUnit=on
      settings: PermitHierarchicalResolution=ParametersOnly
  MATLAB Function4 : Stateflow chart  TreatAsAtomicUnit=on
      settings: PermitHierarchicalResolution=ParametersOnly
  MATLAB Function5 : Stateflow chart  TreatAsAtomicUnit=on
      settings: PermitHierarchicalResolution=ParametersOnly
  MATLAB Function6 : Stateflow chart  TreatAsAtomicUnit=on
      settings: PermitHierarchicalResolution=ParametersOnly
  MATLAB Function7 : Stateflow chart  TreatAsAtomicUnit=on
      settings: PermitHierarchicalResolution=ParametersOnly
  MATLAB Function8 : Stateflow chart  TreatAsAtomicUnit=on
      settings: PermitHierarchicalResolution=ParametersOnly
  Mux : Mux  Inputs=3
  Mux1 : Mux  Inputs=3
  Mux2 : Mux  Inputs=2
  Product{,1,4..9} (8 alike) : Product  Multiplication=Matrix(*)
  Product2 : Product
  Product3 : Product  Inputs=3  Multiplication=Matrix(*)
  Scope : Scope  NumInputPorts=2
      settings: TimeRange=auto  MaxDataPoints=5000  SaveToWorkspace=off  YMin=-10~-5  YMax=10~5  SampleTime=-1
  Sum : Sum  Inputs=-+-++
  Sum1 : Sum  Inputs=|-+
  Sum2 : Sum  Inputs=-+-
  Sum3 : Sum  Inputs=|+-
  Sum4 : Sum  Inputs=|-+
  Sum5 : Sum  Inputs=|++
  Sum6 : Sum  Inputs=|+-
  Sum7 : Sum  Inputs=|+-
  Sum8 : Sum  Inputs=++++
  Sum9 : Sum  Inputs=|-+
  Vector Concatenate : Concatenate  Mode=Multidimensional array
  u : Outport
  wires:
  F/1 -> Vector Concatenate/1  "F1"
  H/1 -> Vector Concatenate/2  "F2"
  p_I/1 -> Sum1/1
  Sum2/1 -> Gain3/1  "z_2"
  Sum1/1 -> Sum/2, Gain1/1, Gain/1  "z_1"
  v_I/1 -> Sum2/2
  Gain/1 -> Sum2/1
  Demux/2 -> Sum2/3  "p_dot_d"
  Demux/3 -> Sum/4  "p_dotdot_d"
  "p_d, p_dot_d, p_dotdot_d"/1 -> Demux/1
  Demux/1 -> Sum1/2  "p_d"
  Sum/1 -> Mux2/1  "u_P"
  Gain1/1 -> Gain2/1
  Gain2/1 -> Sum/1
  Constant/1 -> Sum/5
  Gain3/1 -> Sum/3
  MATLAB Function7/1(q) -> Demux1/1
  Demux1/1 -> Mux/1
  Demux1/2 -> Mux/2
  Demux1/3 -> Mux/3
  Demux1/4 -> MATLAB Function/4(eta)  "eta"
  Mux/1 -> MATLAB Function/3(epsilon)  "epsilon"
  Demux2/2 -> Sum9/2  "omega_dot_d"
  "omega_d, omega_dot_d"/1 -> Demux2/1
  Demux2/1 -> Sum3/1  "omega_d"
  Demux4/3 -> Mux1/3
  MATLAB Function1/1(q) -> Demux4/1
  Demux4/4 -> MATLAB Function/2(eta_d)  "eta_d"
  Demux4/1 -> Mux1/1
  Demux4/2 -> Mux1/2
  Mux1/1 -> MATLAB Function/1(epsilon_d)  "epsilon_d"
  R_d/1 -> MATLAB Function1/1(R)
  Sum3/1 -> MATLAB Function4/5(omega_tilde), Sum4/2, Product/2, Product1/2  "omega_tilde"
  Gain4/1 -> Product/1
  Product/1 -> Integrator/1  "eta_tilde_dot"
  Integrator/1 -> Sum6/1  "eta_tilde"
  Product1/1 -> Gain5/1
  Identity Matrix/1 -> Product2/2
  MATLAB Function/1(eta_tilde) -> MATLAB Function4/6(eta_tilde), MATLAB Function2/1(eta_tilde), MATLAB Function3/1(eta_tilde), Sum6/2, Product2/1  "eta_tilde"
  Product2/1 -> Sum5/1
  MATLAB Function/4(skew_eps_tilde) -> Sum5/2
  Sum5/1 -> Product1/1
  Gain5/1 -> Integrator1/1  "eps_tilde_dot"
  Integrator1/1 -> Sum7/1  "eps_tilde"
  MATLAB Function/2(epsilon_tilde) -> MATLAB Function4/7(eps_tilde), MATLAB Function2/2(eps_tilde), MATLAB Function3/2(eps_tilde), Sum7/2
  Sum7/1 -> Scope/2
  Sum6/1 -> Scope/1
  MATLAB Function/3(epsilon_tilde_T) -> Gain4/1
  Constant1/1 -> Gain6/1, MATLAB Function4/1(K1)
  MATLAB Function3/1(G) -> Product3/2, Product6/1, MATLAB Function4/2(G)
  MATLAB Function2/1(z1) -> Product6/2, MATLAB Function4/3(z1), Product3/3
  Product3/1 -> Sum4/1  "alpha"
  Gain6/1 -> Product3/1
  Sum4/1 -> Product5/2, MATLAB Function4/4(z2)  "z_2"
  MATLAB Function4/1(alpha_dot) -> Sum9/1
  Sum9/1 -> Product4/2
  Constant3/1 -> Product4/1
  Product4/1 -> Sum8/1
  Gain7/1 -> Cross Product1/2
  omega_B/1 -> Gain7/1, Cross Product1/1, Sum3/2  "omega_B"
  Cross Product1/1 -> Sum8/4
  Product5/1 -> Sum8/3
  Constant2/1 -> Product5/1
  Product6/1 -> Sum8/2
  Sum8/1 -> Product9/2  "u_R"
  MATLAB Function5/1(J_inv) -> Product7/1
  Inertia Matrix/1 -> MATLAB Function6/2(I_B)
  Gain8/1 -> MATLAB Function6/1(R_m)
  Vector Concatenate/1 -> Product8/2
  Product7/1 -> u/1
  MATLAB Function6/1(JR) -> Product8/1
  Product8/1 -> MATLAB Function5/1(J)
  R_BtoI/1 -> Gain8/1, MATLAB Function7/1(R)
  Mux2/1 -> Product7/2
  Inertia Matrix1/1 -> MATLAB Function8/1(I)
  MATLAB Function8/1(I_inv) -> Product9/1
  Product9/1 -> Mux2/2

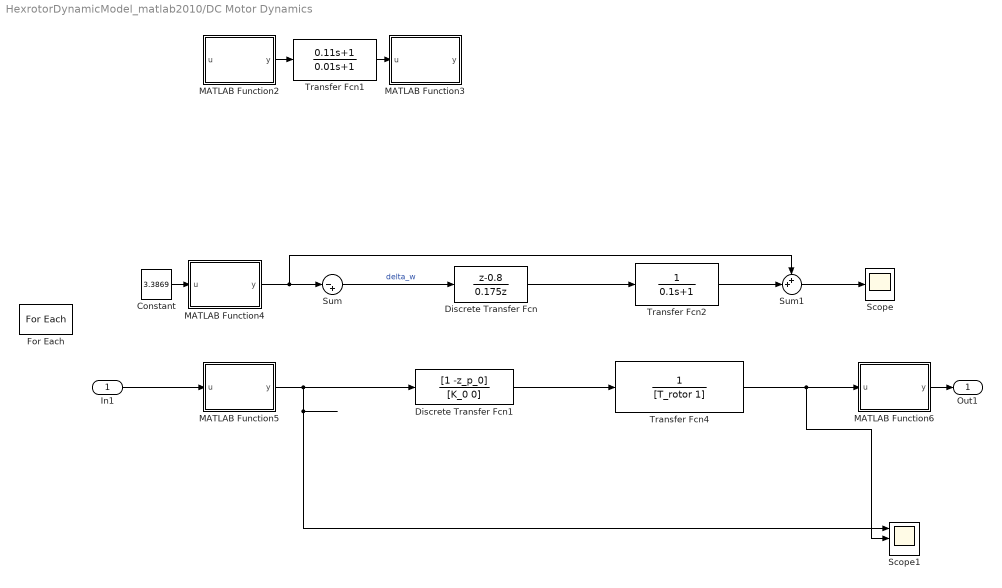
== system HexrotorDynamicModel_matlab2010/DC Motor Dynamics  ==
  In1 : Inport  Partition=on  PartitionDimension=1  PartitionWidth=1
  Constant : Constant  Value=3.3869
  Discrete Transfer Fcn : DiscreteTransferFcn  Numerator=[1 -0.8]  Denominator=[0.175 0]  SampleTime=Ts
  Discrete Transfer Fcn1 : DiscreteTransferFcn  Numerator=[1 -z_p_0]  Denominator=[K_0 0]  InitialStates=274  SampleTime=Ts
  For Each : ForEach  DisableCoverage=on  IndexMode=One-based
  MATLAB Function2 : Stateflow chart  TreatAsAtomicUnit=on
      settings: PermitHierarchicalResolution=ParametersOnly
  MATLAB Function3 : Stateflow chart  TreatAsAtomicUnit=on
      settings: PermitHierarchicalResolution=ParametersOnly
  MATLAB Function4 : Stateflow chart  TreatAsAtomicUnit=on
      settings: PermitHierarchicalResolution=ParametersOnly
  MATLAB Function5 : Stateflow chart  TreatAsAtomicUnit=on  SystemSampleTime=Ts
      settings: PermitHierarchicalResolution=ParametersOnly
  MATLAB Function6 : Stateflow chart  TreatAsAtomicUnit=on
      settings: PermitHierarchicalResolution=ParametersOnly
  Scope : Scope
      settings: TimeRange=auto  MaxDataPoints=5000  SaveToWorkspace=off  YMin=376.971  YMax=680.75438  SampleTime=-1
  Scope1 : Scope  NumInputPorts=3
      settings: TimeRange=auto  MaxDataPoints=5000  SaveToWorkspace=off  SaveName=ScopeData2  YMin=-3413.51419~-5~-5  YMax=3696.18081~5~5  SampleTime=-1
  Sum : Sum  Inputs=|-+
  Sum1 : Sum  Inputs=++|
  Transfer Fcn1 : TransferFcn  Numerator=[0.11 1]  Denominator=[0.01 1]
  Transfer Fcn2 : TransferFcn  Denominator=[0.1 1]
  Transfer Fcn4 : TransferFcn  Denominator=[T_rotor 1]
  Out1 : Outport  ConcatenationDimension=1
  wires:
  Transfer Fcn1/1 -> MATLAB Function3/1(u)
  MATLAB Function2/1(y) -> Transfer Fcn1/1
  Constant/1 -> MATLAB Function4/1(u)
  MATLAB Function4/1(y) -> Sum1/1, Sum/1
  Sum/1 -> Discrete Transfer Fcn/1  "delta_w"
  In1/1 -> MATLAB Function5/1(u)
  MATLAB Function5/1(y) -> Discrete Transfer Fcn1/1, Scope1/1
  Discrete Transfer Fcn/1 -> Transfer Fcn2/1
  Transfer Fcn2/1 -> Sum1/2
  MATLAB Function6/1(y) -> Out1/1
  Sum1/1 -> Scope/1
  Discrete Transfer Fcn1/1 -> Transfer Fcn4/1
  Transfer Fcn4/1 -> Scope1/2, MATLAB Function6/1(u)

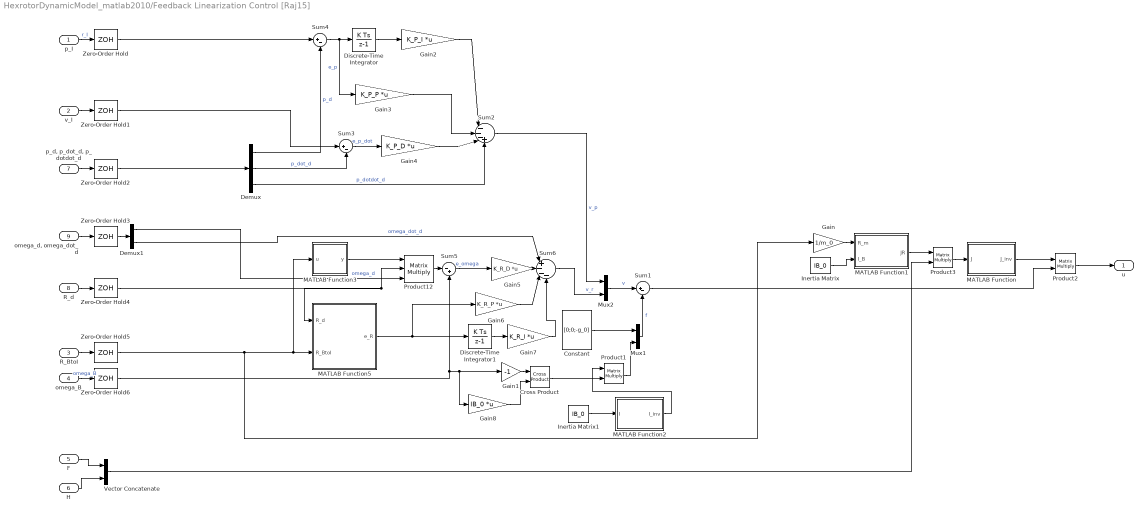
== system HexrotorDynamicModel_matlab2010/Feedback Linearization Control [Raj15] ==
  "p_I " : Inport
  v_I : Inport  Port=2
  "R_BtoI " : Inport  Port=3
  omega_B : Inport  Port=4
  F : Inport  Port=5
  H : Inport  Port=6
  "p_d, p_dot_d, p_dotdot_d" : Inport  Port=7
  R_d : Inport  Port=8
  "omega_d, omega_dot_d" : Inport  Port=9
  Constant : Constant  Value=[0;0;-g_0]  VectorParams1D=off
  Cross Product : vrlib/Utilities/Cross Product
  Demux : Demux  Outputs=3
  Demux1 : Demux  Outputs=2
  Discrete-Time Integrator : DiscreteIntegrator  InitialCondition=[0;0;0]  InitialConditionMode=State only (most efficient)  SampleTime=Ts  ICPrevOutput=DiscIntNeverNeededParam  ICPrevScaledInput=DiscIntNeverNeededParam
  Discrete-Time Integrator1 : DiscreteIntegrator  InitialCondition=[0;0;0]  InitialConditionMode=State only (most efficient)  SampleTime=Ts  ICPrevOutput=DiscIntNeverNeededParam  ICPrevScaledInput=DiscIntNeverNeededParam
  Gain : Gain  Gain=1/m_0
  Gain1 : Gain  Gain=-1
  Gain2 : Gain  Gain=K_P_I  Multiplication=Matrix(K*u)
  Gain3 : Gain  Gain=K_P_P  Multiplication=Matrix(K*u)
  Gain4 : Gain  Gain=K_P_D  Multiplication=Matrix(K*u)
  Gain5 : Gain  Gain=K_R_D  Multiplication=Matrix(K*u)
  Gain6 : Gain  Gain=K_R_P  Multiplication=Matrix(K*u)
  Gain7 : Gain  Gain=K_R_I  Multiplication=Matrix(K*u)
  Gain8 : Gain  Gain=IB_0  Multiplication=Matrix(K*u)
  Inertia Matrix : Constant  Value=IB_0  VectorParams1D=off
  Inertia Matrix1 : Constant  Value=IB_0  VectorParams1D=off
  MATLAB Function : Stateflow chart  TreatAsAtomicUnit=on
      settings: PermitHierarchicalResolution=ParametersOnly
  MATLAB Function1 : Stateflow chart  TreatAsAtomicUnit=on
      settings: PermitHierarchicalResolution=ParametersOnly
  MATLAB Function2 : Stateflow chart  TreatAsAtomicUnit=on
      settings: PermitHierarchicalResolution=ParametersOnly
  MATLAB Function3 : Stateflow chart  TreatAsAtomicUnit=on
      settings: PermitHierarchicalResolution=ParametersOnly
  MATLAB Function5 : Stateflow chart  TreatAsAtomicUnit=on
      settings: PermitHierarchicalResolution=ParametersOnly
  Mux1 : Mux  Inputs=2
  Mux2 : Mux  Inputs=2
  Product1 : Product  Multiplication=Matrix(*)
  Product12 : Product  Inputs=***  Multiplication=Matrix(*)
  Product2 : Product  Multiplication=Matrix(*)
  Product3 : Product  Multiplication=Matrix(*)
  Sum1 : Sum  Inputs=|+-
  Sum2 : Sum  Inputs=|---+
  Sum3 : Sum  Inputs=|+-
  Sum4 : Sum  Inputs=|+-
  Sum5 : Sum  Inputs=|-+
  Sum6 : Sum  Inputs=|+---
  Vector Concatenate : Concatenate  Mode=Multidimensional array
  Zero-Order Hold{,1..6} (7 alike) : ZeroOrderHold  SampleTime=Ts
  u : Outport
  wires:
  Demux/1 -> Sum4/2  "p_d"
  Sum2/1 -> Mux2/1  "v_p"
  Demux/3 -> Sum2/4  "p_dotdot_d"
  "p_I "/1 -> Zero-Order Hold/1  "r_I"
  Gain3/1 -> Sum2/2
  Discrete-Time Integrator/1 -> Gain2/1
  Sum4/1 -> Discrete-Time Integrator/1, Gain3/1  "e_p"
  Demux/2 -> Sum3/2  "p_dot_d"
  v_I/1 -> Zero-Order Hold1/1
  Gain2/1 -> Sum2/1
  Sum3/1 -> Gain4/1  "e_p_dot"
  "p_d, p_dot_d, p_dotdot_d"/1 -> Zero-Order Hold2/1
  Gain4/1 -> Sum2/3
  R_d/1 -> Zero-Order Hold4/1
  Gain5/1 -> Sum6/2
  Gain6/1 -> Sum6/3
  Mux1/1 -> Sum1/2  "f"
  Vector Concatenate/1 -> Product3/2
  Discrete-Time Integrator1/1 -> Gain7/1
  Product3/1 -> MATLAB Function/1(J)
  omega_B/1 -> Zero-Order Hold6/1  "omega_B"
  Constant/1 -> Mux1/1
  Gain/1 -> MATLAB Function1/1(R_m)
  MATLAB Function/1(J_inv) -> Product2/1
  Sum1/1 -> Product2/2
  Gain7/1 -> Sum6/4
  MATLAB Function1/1(JR) -> Product3/1
  Product12/1 -> Sum5/1
  Gain1/1 -> Cross Product/1
  "R_BtoI "/1 -> Zero-Order Hold5/1
  Mux2/1 -> Sum1/1  "v"
  MATLAB Function5/1(e_R) -> Discrete-Time Integrator1/1, Gain6/1
  Inertia Matrix/1 -> MATLAB Function1/2(I_B)
  Sum6/1 -> Mux2/2  "v_r"
  Gain8/1 -> Cross Product/2
  Demux1/2 -> Sum6/1  "omega_dot_d"
  MATLAB Function3/1(y) -> Product12/1
  Demux1/1 -> Product12/3  "omega_d"
  Cross Product/1 -> Product1/2
  Sum5/1 -> Gain5/1  "e_omega"
  F/1 -> Vector Concatenate/1
  H/1 -> Vector Concatenate/2
  "omega_d, omega_dot_d"/1 -> Zero-Order Hold3/1
  Product2/1 -> u/1
  Product1/1 -> Mux1/2
  Inertia Matrix1/1 -> MATLAB Function2/1(I)
  MATLAB Function2/1(I_inv) -> Product1/1
  Zero-Order Hold/1 -> Sum4/1
  Zero-Order Hold1/1 -> Sum3/1
  Zero-Order Hold2/1 -> Demux/1
  Zero-Order Hold3/1 -> Demux1/1
  Zero-Order Hold4/1 -> Product12/2, MATLAB Function5/1(R_d)
  Zero-Order Hold5/1 -> Gain/1, MATLAB Function5/2(R_BtoI), MATLAB Function3/1(u)
  Zero-Order Hold6/1 -> Gain8/1, Gain1/1, Sum5/2

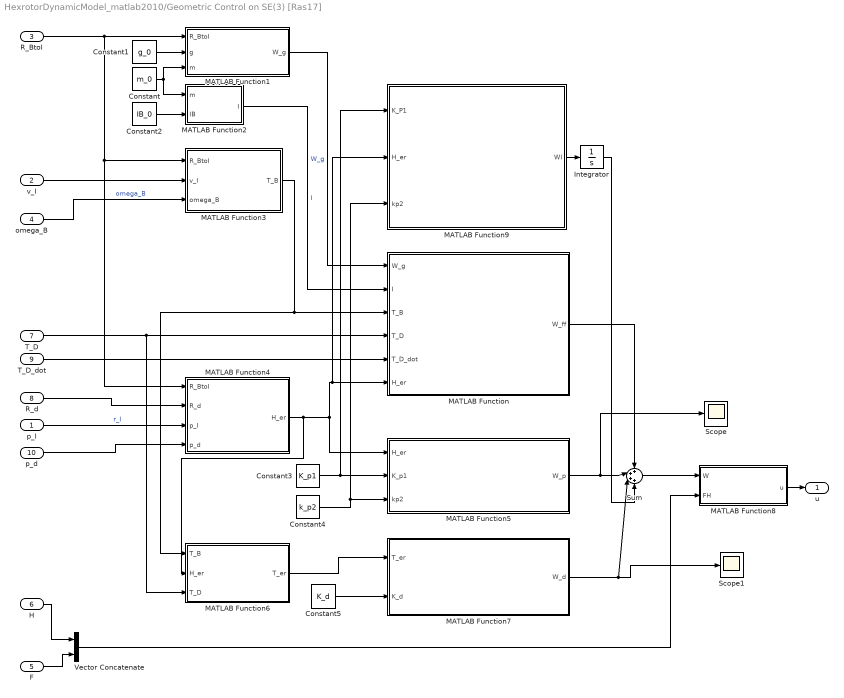
== system HexrotorDynamicModel_matlab2010/Geometric Control on SE(3) [Ras17] ==
  "p_I " : Inport
  v_I : Inport  Port=2
  "R_BtoI " : Inport  Port=3
  omega_B : Inport  Port=4
  F : Inport  Port=5
  H : Inport  Port=6
  T_D : Inport  Port=7
  R_d : Inport  Port=8
  T_D_dot : Inport  Port=9
  p_d : Inport  Port=10
  Constant : Constant  Value=m_0
  Constant1 : Constant  Value=g_0
  Constant2 : Constant  Value=IB_0  VectorParams1D=off
  Constant3 : Constant  Value=K_p1  VectorParams1D=off
  Constant4 : Constant  Value=k_p2
  Constant5 : Constant  Value=K_d  VectorParams1D=off
  Integrator : Integrator  InitialCondition=[0;0;0;0;0;0]
  MATLAB Function : Stateflow chart  TreatAsAtomicUnit=on
      settings: PermitHierarchicalResolution=ParametersOnly
  MATLAB Function1 : Stateflow chart  TreatAsAtomicUnit=on
      settings: PermitHierarchicalResolution=ParametersOnly
  MATLAB Function2 : Stateflow chart  TreatAsAtomicUnit=on
      settings: PermitHierarchicalResolution=ParametersOnly
  MATLAB Function3 : Stateflow chart  TreatAsAtomicUnit=on
      settings: PermitHierarchicalResolution=ParametersOnly
  MATLAB Function4 : Stateflow chart  TreatAsAtomicUnit=on
      settings: PermitHierarchicalResolution=ParametersOnly
  MATLAB Function5 : Stateflow chart  TreatAsAtomicUnit=on
      settings: PermitHierarchicalResolution=ParametersOnly
  MATLAB Function6 : Stateflow chart  TreatAsAtomicUnit=on
      settings: PermitHierarchicalResolution=ParametersOnly
  MATLAB Function7 : Stateflow chart  TreatAsAtomicUnit=on
      settings: PermitHierarchicalResolution=ParametersOnly
  MATLAB Function8 : Stateflow chart  TreatAsAtomicUnit=on
      settings: PermitHierarchicalResolution=ParametersOnly
  MATLAB Function9 : Stateflow chart  TreatAsAtomicUnit=on
      settings: PermitHierarchicalResolution=ParametersOnly
  Scope : Scope
      settings: TimeRange=auto  MaxDataPoints=5000  SaveToWorkspace=off  YMin=-4.41749  YMax=4.33356  SampleTime=-1
  Scope1 : Scope
      settings: TimeRange=auto  MaxDataPoints=5000  SaveToWorkspace=off  SaveName=ScopeData2  YMin=-7.46547  YMax=6.38505  SampleTime=-1
  Sum : Sum  Inputs=++++
  Vector Concatenate : Concatenate  Mode=Multidimensional array
  u : Outport
  wires:
  F/1 -> Vector Concatenate/2
  MATLAB Function1/1(W_g) -> MATLAB Function/1(W_g)  "W_g"
  "R_BtoI "/1 -> MATLAB Function4/1(R_BtoI), MATLAB Function3/1(R_BtoI), MATLAB Function1/1(R_BtoI)
  Constant/1 -> MATLAB Function2/1(m), MATLAB Function1/3(m)
  Constant1/1 -> MATLAB Function1/2(g)
  Constant2/1 -> MATLAB Function2/2(IB)
  MATLAB Function2/1(I) -> MATLAB Function/2(I)  "I"
  MATLAB Function3/1(T_B) -> MATLAB Function6/1(T_B), MATLAB Function/3(T_B)
  v_I/1 -> MATLAB Function3/2(v_I)
  omega_B/1 -> MATLAB Function3/3(omega_B)  "omega_B"
  T_D/1 -> MATLAB Function6/3(T_D), MATLAB Function/4(T_D)
  T_D_dot/1 -> MATLAB Function/5(T_D_dot)
  p_d/1 -> MATLAB Function4/4(p_d)
  "p_I "/1 -> MATLAB Function4/3(p_I)  "r_I"
  R_d/1 -> MATLAB Function4/2(R_d)
  MATLAB Function4/1(H_er) -> MATLAB Function6/2(H_er), MATLAB Function5/1(H_er), MATLAB Function9/2(H_er), MATLAB Function/6(H_er)
  Constant3/1 -> MATLAB Function9/1(K_P1), MATLAB Function5/2(K_p1)
  Constant4/1 -> MATLAB Function9/3(kp2), MATLAB Function5/3(kp2)
  MATLAB Function6/1(T_er) -> MATLAB Function7/1(T_er)
  Constant5/1 -> MATLAB Function7/2(K_d)
  MATLAB Function5/1(W_p) -> Scope/1, Sum/2
  MATLAB Function7/1(W_d) -> Scope1/1, Sum/3
  MATLAB Function/1(W_ff) -> Sum/1
  Vector Concatenate/1 -> MATLAB Function8/2(FH)
  H/1 -> Vector Concatenate/1
  Sum/1 -> MATLAB Function8/1(W)
  MATLAB Function8/1(u) -> u/1
  MATLAB Function9/1(WI) -> Integrator/1
  Integrator/1 -> Sum/4

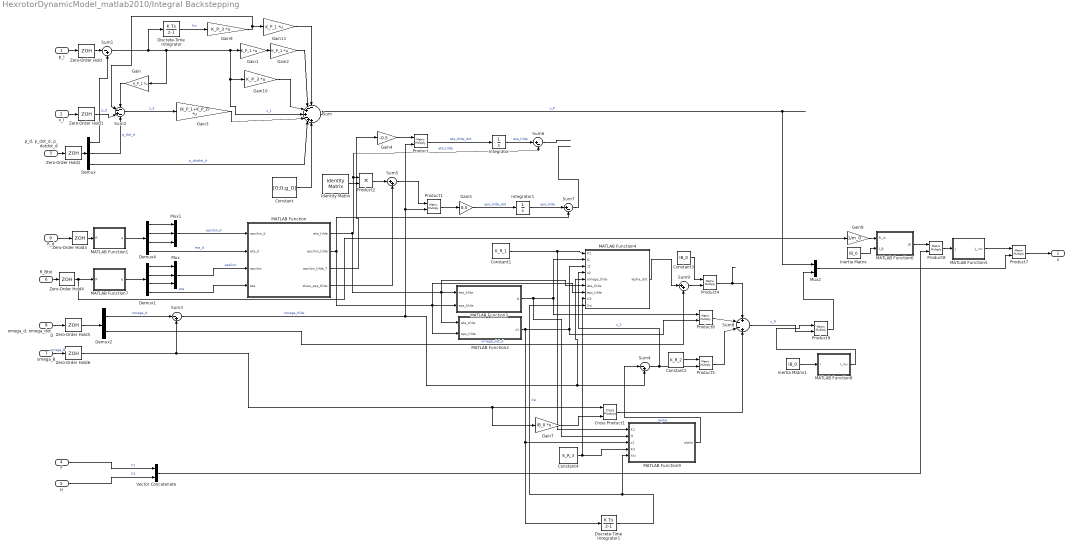
== system HexrotorDynamicModel_matlab2010/Integral Backstepping ==
  p_I : Inport
  v_I : Inport  Port=2
  "p_d, p_dot_d, p_dotdot_d" : Inport  Port=3
  F : Inport  Port=4
  H : Inport  Port=5
  R_BtoI : Inport  Port=6
  omega_B : Inport  Port=7
  "omega_d, omega_dot_d" : Inport  Port=8
  R_d : Inport  Port=9
  Constant : Constant  Value=[0;0;g_0]  VectorParams1D=off
  Constant1 : Constant  Value=K_R_1  VectorParams1D=off
  Constant2 : Constant  Value=K_R_2  VectorParams1D=off
  Constant3 : Constant  Value=IB_0  VectorParams1D=off
  Constant4 : Constant  Value=K_R_3  VectorParams1D=off
  Cross Product1 : vrlib/Utilities/Cross Product
  Demux : Demux  Outputs=3
  Demux1 : Demux
  Demux2 : Demux  Outputs=2
  Demux4 : Demux
  Discrete-Time Integrator : DiscreteIntegrator  InitialCondition=[0;0;0]  InitialConditionMode=State only (most efficient)  SampleTime=Ts  ICPrevOutput=DiscIntNeverNeededParam  ICPrevScaledInput=DiscIntNeverNeededParam
  Discrete-Time Integrator1 : DiscreteIntegrator  InitialCondition=[0;0;0;0]  InitialConditionMode=State only (most efficient)  SampleTime=Ts  ICPrevOutput=DiscIntNeverNeededParam  ICPrevScaledInput=DiscIntNeverNeededParam
  Gain{,1..2,11} (4 alike) : Gain  Gain=K_P_1  Multiplication=Matrix(K*u)
  Gain10 : Gain  Gain=K_P_3  Multiplication=Matrix(K*u)
  Gain3 : Gain  Gain=(K_P_1+K_P_2)  Multiplication=Matrix(K*u)
  Gain4 : Gain  Gain=-0.5
  Gain5 : Gain  Gain=0.5
  Gain7 : Gain  Gain=IB_0  Multiplication=Matrix(K*u)
  Gain8 : Gain  Gain=1/m_0
  Gain9 : Gain  Gain=K_P_3  Multiplication=Matrix(K*u)
  Identity Matrix : dspmtrx3/Identity Matrix  Inherit=off  N=3  Ts=inf  dataType=double  isSigned=on  wordLen=16  udDataType=sfix(16)  fracBitsMode=Best precision  numFracBits=15  OutDataTypeStr=double  LastOutDataTypeStr=double
  Inertia Matrix : Constant  Value=IB_0  VectorParams1D=off
  Inertia Matrix1 : Constant  Value=IB_0  VectorParams1D=off
  Integrator : Integrator  InitialCondition=1
  Integrator1 : Integrator  InitialCondition=[0;0;0]
  MATLAB Function : Stateflow chart  TreatAsAtomicUnit=on
      settings: PermitHierarchicalResolution=ParametersOnly
  MATLAB Function1 : Stateflow chart  TreatAsAtomicUnit=on
      settings: PermitHierarchicalResolution=ParametersOnly
  MATLAB Function2 : Stateflow chart  TreatAsAtomicUnit=on
      settings: PermitHierarchicalResolution=ParametersOnly
  MATLAB Function3 : Stateflow chart  TreatAsAtomicUnit=on
      settings: PermitHierarchicalResolution=ParametersOnly
  MATLAB Function4 : Stateflow chart  TreatAsAtomicUnit=on
      settings: PermitHierarchicalResolution=ParametersOnly
  MATLAB Function5 : Stateflow chart  TreatAsAtomicUnit=on
      settings: PermitHierarchicalResolution=ParametersOnly
  MATLAB Function6 : Stateflow chart  TreatAsAtomicUnit=on
      settings: PermitHierarchicalResolution=ParametersOnly
  MATLAB Function7 : Stateflow chart  TreatAsAtomicUnit=on
      settings: PermitHierarchicalResolution=ParametersOnly
  MATLAB Function8 : Stateflow chart  TreatAsAtomicUnit=on
      settings: PermitHierarchicalResolution=ParametersOnly
  MATLAB Function9 : Stateflow chart  TreatAsAtomicUnit=on
      settings: PermitHierarchicalResolution=ParametersOnly
  Mux : Mux  Inputs=3
  Mux1 : Mux  Inputs=3
  Mux2 : Mux  Inputs=2
  Product{,1,4..9} (8 alike) : Product  Multiplication=Matrix(*)
  Product2 : Product
  Sum : Sum  Inputs=--++-++
  Sum1 : Sum  Inputs=|-+
  Sum2 : Sum  Inputs=--+-
  Sum3 : Sum  Inputs=|-+
  Sum4 : Sum  Inputs=|-+
  Sum5 : Sum  Inputs=|++
  Sum6 : Sum  Inputs=|+-
  Sum7 : Sum  Inputs=|+-
  Sum8 : Sum  Inputs=+--+
  Sum9 : Sum  Inputs=|++
  Vector Concatenate : Concatenate  Mode=Multidimensional array
  Zero-Order Hold{,1..6} (7 alike) : ZeroOrderHold  SampleTime=Ts
  u : Outport
  wires:
  F/1 -> Vector Concatenate/1  "F1"
  H/1 -> Vector Concatenate/2  "F2"
  p_I/1 -> Zero-Order Hold/1
  Sum2/1 -> Gain3/1  "z_2"
  Sum1/1 -> Discrete-Time Integrator/1, Sum/4, Gain10/1, Gain1/1, Gain/1  "z_1"
  v_I/1 -> Zero-Order Hold1/1
  Gain/1 -> Sum2/1
  Demux/2 -> Sum2/4  "p_dot_d"
  Demux/3 -> Sum/6  "p_dotdot_d"
  "p_d, p_dot_d, p_dotdot_d"/1 -> Zero-Order Hold2/1
  Demux/1 -> Sum1/2  "p_d"
  Sum/1 -> Mux2/1  "u_P"
  Gain1/1 -> Gain2/1
  Gain2/1 -> Sum/2
  Constant/1 -> Sum/7
  Gain3/1 -> Sum/5
  MATLAB Function7/1(q) -> Demux1/1
  Demux1/1 -> Mux/1
  Demux1/2 -> Mux/2
  Demux1/3 -> Mux/3
  Demux1/4 -> MATLAB Function/4(eta)  "eta"
  Mux/1 -> MATLAB Function/3(epsilon)  "epsilon"
  Demux2/2 -> Sum9/2  "omega_dot_d"
  "omega_d, omega_dot_d"/1 -> Zero-Order Hold5/1
  Demux2/1 -> Sum3/1  "omega_d"
  Demux4/3 -> Mux1/3
  MATLAB Function1/1(q) -> Demux4/1
  Demux4/4 -> MATLAB Function/2(eta_d)  "eta_d"
  Demux4/1 -> Mux1/1
  Demux4/2 -> Mux1/2
  Mux1/1 -> MATLAB Function/1(epsilon_d)  "epsilon_d"
  Zero-Order Hold3/1 -> MATLAB Function1/1(R)
  Sum3/1 -> MATLAB Function4/5(omega_tilde), Sum4/2, Product/2, Product1/2  "omega_tilde"
  Gain4/1 -> Product/1
  Product/1 -> Integrator/1  "eta_tilde_dot"
  Integrator/1 -> Sum6/1  "eta_tilde"
  Product1/1 -> Gain5/1
  Identity Matrix/1 -> Product2/2
  MATLAB Function/1(eta_tilde) -> MATLAB Function4/6(eta_tilde), MATLAB Function2/1(eta_tilde), MATLAB Function3/1(eta_tilde), Sum6/2, Product2/1  "eta_tilde"
  Product2/1 -> Sum5/1
  MATLAB Function/4(skew_eps_tilde) -> Sum5/2
  Sum5/1 -> Product1/1
  Gain5/1 -> Integrator1/1  "eps_tilde_dot"
  Integrator1/1 -> Sum7/1  "eps_tilde"
  MATLAB Function/2(epsilon_tilde) -> MATLAB Function4/7(eps_tilde), MATLAB Function2/2(eps_tilde), MATLAB Function3/2(eps_tilde), Sum7/2
  Sum7/1 -> ?
  Sum6/1 -> ?
  MATLAB Function/3(epsilon_tilde_T) -> Gain4/1
  Constant1/1 -> MATLAB Function9/1(K1), MATLAB Function4/1(K1)
  MATLAB Function3/1(G) -> MATLAB Function9/2(G), Product6/1, MATLAB Function4/2(G)
  MATLAB Function2/1(z1) -> Product6/2, MATLAB Function4/3(z1), MATLAB Function9/3(z1), Discrete-Time Integrator1/1
  MATLAB Function9/1(alpha) -> Sum4/1  "alpha"
  Sum4/1 -> Product5/2, MATLAB Function4/4(z2)  "z_2"
  MATLAB Function4/1(alpha_dot) -> Sum9/1
  Sum9/1 -> Product4/2
  Constant3/1 -> Product4/1
  Product4/1 -> Sum8/1
  Gain7/1 -> Cross Product1/2
  omega_B/1 -> Zero-Order Hold6/1  "omega_B"
  Cross Product1/1 -> Sum8/4
  Product5/1 -> Sum8/3
  Constant2/1 -> Product5/1
  Product6/1 -> Sum8/2
  Sum8/1 -> Product9/2  "u_R"
  MATLAB Function5/1(J_inv) -> Product7/1
  Inertia Matrix/1 -> MATLAB Function6/2(I_B)
  Gain8/1 -> MATLAB Function6/1(R_m)
  Vector Concatenate/1 -> Product8/2
  Product7/1 -> u/1
  MATLAB Function6/1(JR) -> Product8/1
  Product8/1 -> MATLAB Function5/1(J)
  Zero-Order Hold4/1 -> Gain8/1, MATLAB Function7/1(R)
  Mux2/1 -> Product7/2
  Inertia Matrix1/1 -> MATLAB Function8/1(I)
  MATLAB Function8/1(I_inv) -> Product9/1
  Product9/1 -> Mux2/2
  Discrete-Time Integrator/1 -> Gain9/1  "Xsi"
  Gain9/1 -> Gain11/1, Sum2/2
  Gain10/1 -> Sum/3
  Gain11/1 -> Sum/1
  Discrete-Time Integrator1/1 -> MATLAB Function4/9(Xsi), MATLAB Function9/5(Xsi)  "Xsi"
  Constant4/1 -> MATLAB Function9/4(K3), MATLAB Function4/8(K3)
  Zero-Order Hold/1 -> Sum1/1
  Zero-Order Hold1/1 -> Sum2/3
  Zero-Order Hold2/1 -> Demux/1
  R_d/1 -> Zero-Order Hold3/1
  R_BtoI/1 -> Zero-Order Hold4/1
  Zero-Order Hold5/1 -> Demux2/1
  Zero-Order Hold6/1 -> Gain7/1, Cross Product1/1, Sum3/2
